simulink model "Zaehler"  (R2022a)
settings: Solver=ode3  StartTime=0.0  StopTime=10.0  FixedStep=0.01  RelTol=1e-3  EnableMultiTasking=on
settings Model: Creator=60251  LastModifiedBy=yufu
settings SolverCC: AlgebraicLoopSolver=TrustRegion
settings DebuggingCC: UnconnectedInputMsg=warning  UnconnectedOutputMsg=warning  UnconnectedLineMsg=warning  SFMachineParentedDataDiag=warning
settings RTWCC: DLArmComputeVersion=19.05

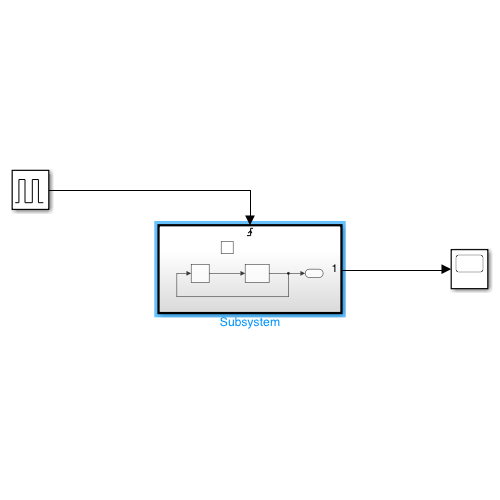
[thumbnail: Simulink's stored preview of the top-level diagram]
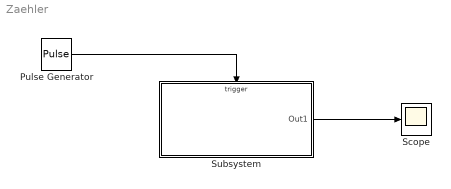
== system Zaehler ==
  Pulse Generator : DiscretePulseGenerator  PulseType=Time based  PulseWidth=50
  Scope : Scope
  Subsystem : Subsystem
  wires:
  Pulse Generator/1 -> Subsystem/Trigger
  Subsystem/1(Out1) -> Scope/1

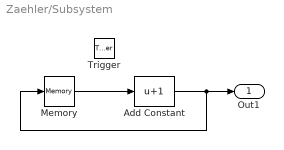
== system Zaehler/Subsystem ==
  Trigger : TriggerPort  VariantControl=Variant  PortDimensions=1
  Add Constant : Bias  Bias=1  SaturateOnIntegerOverflow=off
  Memory : Memory  InheritSampleTime=on
  Out1 : Outport
  wires:
  Memory/1 -> Add Constant/1
  Add Constant/1 -> Memory/1, Out1/1
